simulink model "logitudional_teste"  (R2024b)
settings: Solver=ode4  StartTime=0.0  StopTime=80  FixedStep=1e-3  RelTol=1e-3
undefined symbols (not defined in the file): d_gain, distancia_eixo_ftraseiro_centro_massa, filtro_coeficiente, i_gain, massa, p_gain
libraries: slpidlib x1, autolibshared x1
settings Model: DataDictionary=modelo_bike_r23a.sldd  Creator=thailon  LastModifiedBy=lucas
settings RTWCC: GPUComputeCapability=3.5

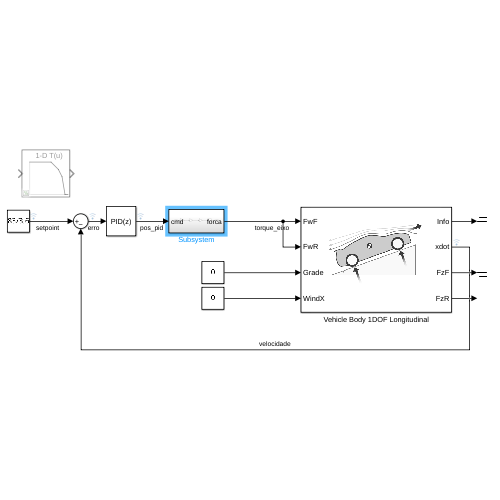
[thumbnail: Simulink's stored preview of the top-level diagram]
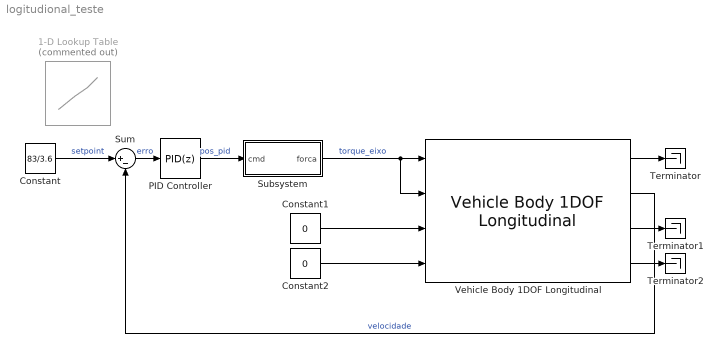
== system logitudional_teste ==
  1-D Lookup Table : Lookup_n-D  Commented=on  NumberOfTableDimensions=1  BreakpointsForDimension1=[0 11200 15000 17000 18700 20000]  Table=[29.1 29.1 26.6 24 18 18]  InternalRulePriority=Speed  RndMeth=Simplest
  Constant : Constant  Value=83/3.6
  Constant1 : Constant  Value=0
  Constant2 : Constant  Value=0
  PID Controller : slpidlib/PID Controller  Controller=PID  Form=Parallel  TimeDomain=Discrete-time  UseExternalTs=off  SampleTime=-1  IntegratorMethod=Forward Euler  FilterMethod=Forward Euler  ControllerParametersSource=internal  P=p_gain  I=i_gain  UseKiTs=off  D=d_gain  UseExternalDerivativeSource=off  N=filtro_coeficiente  UseFilter=on  TunerSelectOption=Transfer Function Based (PID Tuner App)  InitialConditionSource=internal  InitialConditionForIntegrator=0  InitialConditionForFilter=0  DifferentiatorICPrevScaledInput=0  ExternalReset=none  TrackingMode=off  Kt=1  LimitOutput=off  SatLimitsSource=internal  UpperSaturationLimit=inf  LowerSaturationLimit=-inf  LinearizeAsGain=on  AntiWindupMode=none  Kb=1  LimitIntegrator=off  UpperIntegratorSaturationLimit=inf  LowerIntegratorSaturationLimit=-inf  POutMin=[]  POutMax=[]  IOutMin=[]  IOutMax=[]  DOutMin=[]  DOutMax=[]  NOutMin=[]  NOutMax=[]  SumOutMin=[]  SumOutMax=[]  SaturationOutMin=[]  SaturationOutMax=[]  PParamMin=[]  PParamMax=[]  IParamMin=[]  IParamMax=[]  DParamMin=[]  DParamMax=[]  NParamMin=[]  NParamMax=[]  KbParamMin=[]  KbParamMax=[]  KtParamMin=[]  KtParamMax=[]  KbOutMin=[]  KbOutMax=[]  KtOutMin=[]  KtOutMax=[]  IntegratorOutMin=[]  IntegratorOutMax=[]  FilterOutMin=[]  FilterOutMax=[]  SumI1OutMin=[]  SumI1OutMax=[]  SumI2OutMin=[]  SumI2OutMax=[]  SumI3OutMin=[]  SumI3OutMax=[]  SumI4OutMin=[]  SumI4OutMax=[]  SumDOutMin=[]  SumDOutMax=[]  DifferentiatorOutMin=[]  DifferentiatorOutMax=[]  FilterDiffOutCoefMin=[]  FilterDiffOutCoefMax=[]  ReciprocalOutMin=[]  ReciprocalOutMax=[]  SumDenOutMin=[]  SumDenOutMax=[]  SumNumOutMin=[]  SumNumOutMax=[]  DivideOutMin=[]  DivideOutMax=[]  UdiffTsProdOutMin=[]  UdiffTsProdOutMax=[]  NTsProdOutMin=[]  NTsProdOutMax=[]  UintegralTsProdOutMin=[]  UintegralTsProdOutMax=[]  UngainTsProdOutMin=[]  UngainTsProdOutMax=[]  ClampingZeroOutDataTypeStr=Inherit: Inherit via back propagation  ClampingZeroOutMin=[]  ClampingZeroOutMax=[]  FilterDenConstantOutDataTypeStr=Inherit: Inherit via back propagation  FilterDenConstantOutMin=[]  FilterDenConstantOutMax=[]  PCopyOutDataTypeStr=Inherit: Inherit via back propagation  PCopyOutMin=[]  PCopyOutMax=[]  NCopyOutDataTypeStr=Inherit: Inherit via back propagation  NCopyOutMin=[]  NCopyOutMax=[]  IntegratorContinuousStateAttributes=''  IntegratorStateMustResolveToSignalObject=off  IntegratorRTWStateStorageClass=Auto  FilterContinuousStateAttributes=''  FilterStateMustResolveToSignalObject=off  FilterRTWStateStorageClass=Auto  ParallelPVariant=InternalParameters  IdealPVariant=Disabled  IVariant=InternalParameters  DVariant=InternalParameters  IntegratorVariant=Discrete  SatVariant=Disabled  AWVariant=Passthrough  PCopyVariant=Disabled  TRVariant=Disabled  FdbkBlocksVariant=Forward  IdealPFdbkVariant=Disabled  SatFdbkVariant=Disabled  DerivativeFilterVariant=ForwardEulerFilter  NVariant=InternalParameters  NCopyVariant=Disabled  FilterICVariant=InternalICsFilter  IntegratorICVariant=InternalICs  ExternalResetVariant=Disabled  TRSumVariant=Passthrough  SumFdbkVariant=Disabled  SumVariant=Sum_PID  TsampFilterVariant=InternalTs  TsampNgainVariant=Passthrough  TsampIntegralVariant=Disabled_SignalSpec  ExternalSaturationOutDataTypeStr=Inherit: Same as second input  DerivativeSourceVariant=ErrorSignal  PreIntVariant=InternalPreInt
  Subsystem : Subsystem
  Sum : Sum  Inputs=|+-
  Terminator : Terminator
  Terminator1 : Terminator
  Terminator2 : Terminator
  Vehicle Body 1DOF Longitudinal : autolibshared/Vehicle Body 1DOF Longitudinal  VariantControl=SL  extFMode=off  extMMode=off  extTamb=off  wind3D=off  aMode=1  NF=numero_de_eixos_frente  NR=numero_de_eixos_traseira  m=massa  a=distancia_eixo_frontal_centro_massa  b=distancia_eixo_ftraseiro_centro_massa  h=distancia_chao_plano_centro_massa  Cd=coeficiente_longitudinal_arrasto  Cl=coefficient_longitudinal_sustentacao  Cpm=arrasto_longitudinal_pitch  Af=area_arrasto_longitudinal  x_o=0  xdot_o=velocidade_inicial  Pabs=101325  T=273  g=9.81
      settings: LibrarySourceBlock=autolibvehdynlong/Vehicle Body 1DOF Longitudinal
  wires:
  Constant/1 -> Sum/1  "setpoint"
  Vehicle Body 1DOF Longitudinal/2 -> Sum/2  "velocidade"
  Subsystem/1(forca) -> Vehicle Body 1DOF Longitudinal/2, Vehicle Body 1DOF Longitudinal/1  "torque_eixo"
  Constant1/1 -> Vehicle Body 1DOF Longitudinal/3
  Constant2/1 -> Vehicle Body 1DOF Longitudinal/4
  Vehicle Body 1DOF Longitudinal/1 -> Terminator/1
  Vehicle Body 1DOF Longitudinal/3 -> Terminator1/1
  Vehicle Body 1DOF Longitudinal/4 -> Terminator2/1
  Sum/1 -> PID Controller/1  "erro"
  PID Controller/1 -> Subsystem/1(cmd)  "pos_pid"

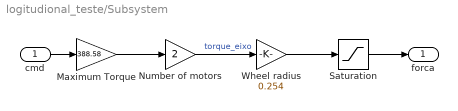
== system logitudional_teste/Subsystem ==
  cmd : Inport
  Maximum Torque : Gain  Gain=388.58
  Number of motors : Gain  Gain=2
  Saturation : Saturate  UpperLimit=1147.77  LowerLimit=0
  Wheel radius : Gain  Gain=0.254
  forca : Outport
  wires:
  Saturation/1 -> forca/1
  Wheel radius/1 -> Saturation/1
  Number of motors/1 -> Wheel radius/1  "torque_eixo"
  Maximum Torque/1 -> Number of motors/1
  cmd/1 -> Maximum Torque/1
